simulink model "my_buck_nn_3_30"  (R2021a)
settings: Solver=ode8  StartTime=0.0  StopTime=T  RelTol=1e-3  EnableMultiTasking=on
undefined symbols (not defined in the file): a00c, a00o, a01c, a01o, a10c, a10o, a11c, a11o, b0c, b0o, b1c, b1o, i0, T_sw, v0
libraries: neural x95, simulink x1
(part 5 of 5)

== system my_buck_nn_3_30/Feed-Forward Neural Network/Layer 4/Delays 1 ==
  "p{4}" : Inport  PortDimensions=30
      mask Display: e = 0.06;c1 = [120 230 180]/255;c2 = ([120 230 180]+0)/(256+128);c3 = ([120 230 180]+128)/(256+128);patch([0 1 1 0],[0 0 1 1],c1);patch([0 1 1 1-e 1-e 0+e],[0 0 1 1-e 0+e 0+e],c2);patch([0 0 1 1-e 0+e 0+e],[0 1 1 1-e 1-e 0+e],c3);plot([0 1 1 0 0],[0 0 1 1 0]);
  mux : Mux  Inputs=1
      mask Display: e = 0.06;c1 = [120 150 230]/255;c2 = ([120 150 230]+0)/383;c3 = ([120 150 230]+128)/383;patch([0 1 1 0],[0 0 1 1],c1);patch([0 1 1 1-e 1-e 0+e],[0 0 1 1-e 0+e 0+e],c2);patch([0 0 1 1-e 0+e 0+e],[0 1 1 1-e 1-e 0+e],c3);plot([0 1 1 0 0],[0 0 1 1 0]);disp('Mux')
  "pd{4,3}" : Outport
      mask Display: e = 0.06;c1 = [120 230 180]/255;c2 = ([120 230 180]+0)/(256+128);c3 = ([120 230 180]+128)/(256+128);patch([0 1 1 0],[0 0 1 1],c1);patch([0 1 1 1-e 1-e 0+e],[0 0 1 1-e 0+e 0+e],c2);patch([0 0 1 1-e 0+e 0+e],[0 1 1 1-e 1-e 0+e],c3);plot([0 1 1 0 0],[0 0 1 1 0]);
  wires:
  "p{4}"/1 -> mux/1
  mux/1 -> "pd{4,3}"/1

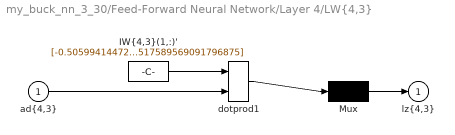
== system my_buck_nn_3_30/Feed-Forward Neural Network/Layer 4/LW{4,3} ==
  "ad{4,3}" : Inport  PortDimensions=30
      mask Display: e = 0.06;c1 = [120 230 180]/255;c2 = ([120 230 180]+0)/(256+128);c3 = ([120 230 180]+128)/(256+128);patch([0 1 1 0],[0 0 1 1],c1);patch([0 1 1 1-e 1-e 0+e],[0 0 1 1-e 0+e 0+e],c2);patch([0 0 1 1-e 0+e 0+e],[0 1 1 1-e 1-e 0+e],c3);plot([0 1 1 0 0],[0 0 1 1 0]);
  "IW{4,3}(1,:)'" : Constant  Value=[-0.5059941447269509229300865627010352909564971923828125;0.8241308777514058103719207792892120778560638427734375;-0.4392503016426159145879637435427866876125335693359375;-0.811835195686756438959719162085093557834625244140625;-0.08879518823044418862622251253924332559108734130859375;0.436170778543745141231369188972166739404201507568359375;-0.372836477249718800663913498283363878726959228515625;0.49327925464464161819932996877469122409820556640625;-1.1600297042505400835210593868396244943141937255859375;-0.10989545034795099309743449111920199356973171234130859375;-0.31788999776713888767432081294828094542026519775390625;-0.51107337769876048927386591458343900740146636962890625;0.060475104713252958443803208865574561059474945068359375;1.00480041786385410063076051301322877407073974609375;-0.1387172485603772875695227639880613423883914947509765625;0.460988389165658707380401892805821262300014495849609375;0.2458079369223395982402280424139462411403656005859375;-0.59467887402099339766436969512142241001129150390625;0.82307383045923432351997917066910304129123687744140625;0.3840871320221255214022448853938840329647064208984375;0.86921731920315570274482297463691793382167816162109375;0.66962628874172247517293499186052940785884857177734375;0.047214237730998191711062617059724288992583751678466796875;0.0252735621813702550364499899160364293493330478668212890625;0.76617982867512235412021937008830718696117401123046875;-0.773650511837385312929882275057025253772735595703125;0.10390922538583773071518834285598131828010082244873046875;-0.811717029993660244002740000723861157894134521484375;-0.67759022605497687408160345512442290782928466796875;0.1029170557705458566299938638621824793517589569091796875]
      mask Display: e = 0.06;c1 = [120 150 230]/255;c2 = ([120 150 230]+0)/383;c3 = ([120 150 230]+128)/383;patch([0 1 1 0],[0 0 1 1],c1);patch([0 1 1 1-e 1-e 0+e],[0 0 1 1-e 0+e 0+e],c2);patch([0 0 1 1-e 0+e 0+e],[0 1 1 1-e 1-e 0+e],c3);plot([0 1 1 0 0],[0 0 1 1 0]);disp('weights');
  Mux : Mux  Inputs=1
      mask Display: e = 0.06;c1 = [120 150 230]/255;c2 = ([120 150 230]+0)/383;c3 = ([120 150 230]+128)/383;patch([0 1 1 0],[0 0 1 1],c1);patch([0 1 1 1-e 1-e 0+e],[0 0 1 1-e 0+e 0+e],c2);patch([0 0 1 1-e 0+e 0+e],[0 1 1 1-e 1-e 0+e],c3);plot([0 1 1 0 0],[0 0 1 1 0]);disp('Mux');
  dotprod1 : neural/Weight Functions/dotprod
  "lz{4,3}" : Outport
      mask Display: e = 0.06;c1 = [120 230 180]/255;c2 = ([120 230 180]+0)/(256+128);c3 = ([120 230 180]+128)/(256+128);patch([0 1 1 0],[0 0 1 1],c1);patch([0 1 1 1-e 1-e 0+e],[0 0 1 1-e 0+e 0+e],c2);patch([0 0 1 1-e 0+e 0+e],[0 1 1 1-e 1-e 0+e],c3);plot([0 1 1 0 0],[0 0 1 1 0]);
  wires:
  "IW{4,3}(1,:)'"/1 -> dotprod1/1
  "ad{4,3}"/1 -> dotprod1/2
  dotprod1/1 -> Mux/1
  Mux/1 -> "lz{4,3}"/1

== stateflow chart my_buck_nn_3_30/Buck Converter ==
  settings: updateMethod=CONTINUOUS
  state Discontinuous
    du:
    i_dot = 0;
    v_dot = a11o*v+b1o;
    t_dot = 1;
    i_out = i;
    v_out = v;
    mode_out=3;
  state Charging
    du:
    i_dot = a00c*i+a01c*v+b0c;
    v_dot = a10c*i+a11c*v+b1c;
    t_dot = 1;
    i_out = i;
    v_out = v;
    mode_out=2;
  state Discharging
    du:
    i_dot = a00o*i+a01o*v+b0o;
    v_dot = a10o*i+a11o*v+b1o;
    t_dot = 1;
    i_out = i;
    v_out = v;
    mode_out=1;
  Discharging -> Discontinuous [order 2] : [i < 0]
  Discontinuous -> Charging : [mode >= 1]
      | {t = 0;}
  Charging -> Discharging : [mode < 1]
  Discharging -> Charging [order 1] : [mode >= 1]
      | {t = 0;}
  (default) -> Charging : {i = i0;
      | v = v0;}
  data: t local double; i_out output double; v_out output double; i local double; a00o local double =a00o; a01o local double =a01o; a10o local double =a10o; a11o local double =a11o; a00c local double =a00c; a01c local double =a01c; a10c local double =a10c; a11c local double =a11c; b0o local double =b0o; b1o local double =b1o; b0c local double =b0c; b1c local double =b1c; v local double; i0 input double; v0 input double; mode input double =120; mode_out output double
  data t settings: updateMethod=SF_CONTINUOUS_TIME_DATA
  data i settings: updateMethod=SF_CONTINUOUS_TIME_DATA
  data v settings: updateMethod=SF_CONTINUOUS_TIME_DATA
